simulink model "zad3"  (R2018b)
settings: Solver=VariableStepAuto  StartTime=0.0  StopTime=50.0  RelTol=1e-3
values from neighbouring files (symbols this model uses):
  A = 1    [skrypt1.m]    (also in skrypt3.m = 4)
  D = [2 0.1 1]    [skrypt3.m]
  f = 60    [skrypt1.m]    (also in skrypt3.m = 5; skrypt4.m = 17.359375)
  p = -3    [skrypt1.m]    (also in skrypt3.m = 0)
  U = [1]    [skrypt3.m]
settings Model: Creator=hubert  LastModifiedBy=hubert

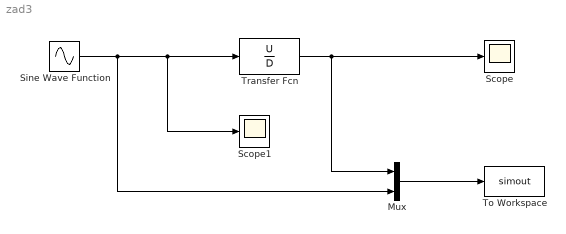
== system zad3 ==
  Mux : Mux  Inputs=2
  Scope : Scope
  Scope1 : Scope
  Sine Wave Function : Sin  Amplitude=A  Frequency=f  Phase=p  SampleTime=0
  To Workspace : ToWorkspace  VariableName=simout  SaveFormat=Timeseries  SampleTime=-1
  Transfer Fcn : TransferFcn  Numerator=U  Denominator=D
  wires:
  Sine Wave Function/1 -> Mux/2, Scope1/1, Transfer Fcn/1
  Transfer Fcn/1 -> Mux/1, Scope/1
  Mux/1 -> To Workspace/1
